simulink model "cartesian_trajectory_planner"  (R2020a)
settings: Solver=ode3  StartTime=0.0  StopTime=10  FixedStep=0.05  RelTol=1e-3
libraries: robotcorelib x2, robotmaniplib x2, simulink x1
settings Model: Creator=paolo  LastModifiedBy=paolo
settings OptimizationCC: EnhancedBackFolding=on  PassReuseOutputArgsAs=Individual arguments  ZeroExternalMemoryAtStartup=off  ZeroInternalMemoryAtStartup=off  MaxStackSize=64  OptimizeBlockOrder=speed  DifferentSizesBufferReuse=on  OptimizationCustomize=off  EfficientTunableParamExpr=on
settings DebuggingCC: ParameterTunabilityLossMsg=error
settings HardwareCC: ProdBitPerPointer=32  ProdBitPerSizeT=32  ProdBitPerPtrDiffT=32  ProdLargestAtomicFloat=None  ProdIntDivRoundTo=Undefined  ProdEndianess=Unspecified  ProdWordSize=32  ProdHWDeviceType=Generic->Unspecified (assume 32-bit Generic)
settings SFSimCC: MATLABDynamicMemAlloc=off
settings RTWCC: SystemTargetFile=ert.tlc  HardwareBoard=Robot Operating System (ROS)  TemplateMakefile=ert_default_tmf  Toolchain=Catkin  TargetLang=C++
settings CodeAppCC: ForceParamTrailComments=on  IgnoreCustomStorageClasses=off  OperatorAnnotations=on  SimulinkDataObjDesc=on  SFDataObjDesc=on  InsertBlockDesc=on

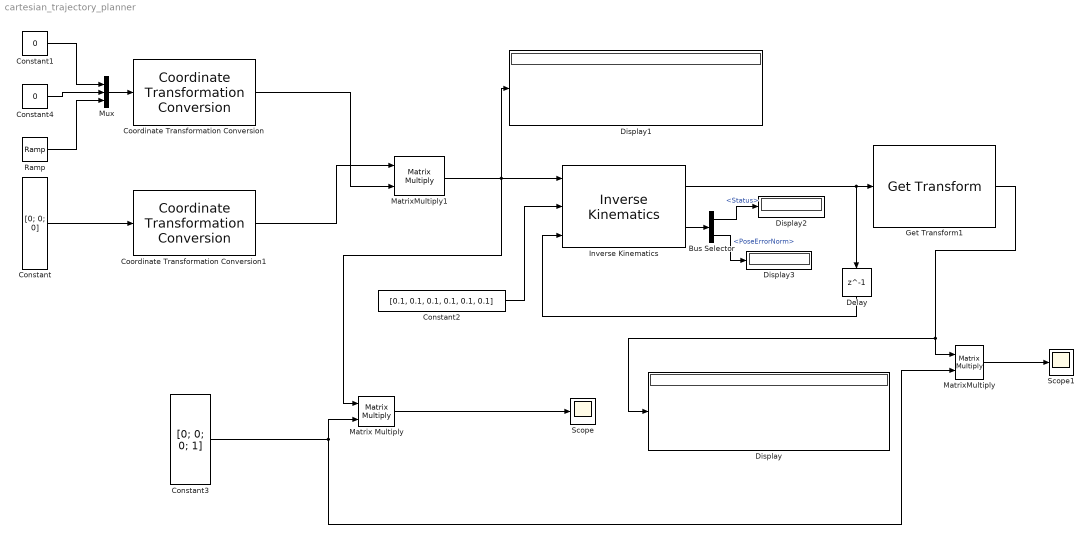
== system cartesian_trajectory_planner ==
  Bus Selector : BusSelector  OutputSignals=Status,PoseErrorNorm
  Constant : Constant  Value=[0; 0; 0]  VectorParams1D=off
  Constant1 : Constant  Value=0
  Constant2 : Constant  Value=[0.1, 0.1, 0.1, 0.1, 0.1, 0.1]
  Constant3 : Constant  Value=[0; 0; 0; 1]  VectorParams1D=off
  Constant4 : Constant  Value=0
  Coordinate Transformation Conversion : robotcorelib/Coordinate Transformation Conversion  InputRepresentation=Translation Vector  InputEulerSequence=ZYX  ShowTrVecInputPort=on  OutputRepresentation=Homogeneous Transformation  OutputEulerSequence=ZYX  ShowTrVecOutputPort=on  SimulateUsing=Interpreted execution
      settings: SourceProductBaseCode=NV,RO,RR
  Coordinate Transformation Conversion1 : robotcorelib/Coordinate Transformation Conversion  InputRepresentation=Euler Angles  InputEulerSequence=XYZ  ShowTrVecInputPort=off  OutputRepresentation=Homogeneous Transformation  OutputEulerSequence=ZYX  ShowTrVecOutputPort=on  SimulateUsing=Interpreted execution
      settings: SourceProductBaseCode=NV,RO,RR
  Delay : Delay  DelayLength=1  InitialCondition=[0; 0; 0; 0; 0; 0]
  Display{,1..3} (4 alike) : Display
  Get Transform1 : robotmaniplib/Get Transform  RigidBodyTree=robot  SourceBody=edo_link_ee  TargetBody=world  SimulateUsing=Interpreted execution
  Inverse Kinematics : robotmaniplib/Inverse Kinematics  RigidBodyTree=robot  EndEffector=edo_link_ee  ShowInfo=on  SolverName=BFGS Gradient Projection  EnforceJointLimits=on  MaxIterations=1500  MaxTime=10  GradientTolerance=1e-7  SolutionTolerance=1e-6  StepTolerance=1e-14  ErrorChangeTolerance=1e-12  UseErrorDamping=on  DampingBias=0.0025  SimulateUsing=Interpreted execution
  Matrix Multiply : Product  Multiplication=Matrix(*)
  MatrixMultiply : Product  Multiplication=Matrix(*)
  MatrixMultiply1 : Product  Multiplication=Matrix(*)
  Mux : Mux  Inputs=3
  Ramp : simulink/Sources/Ramp  slope=-0.01  start=0  InitialOutput=0.99
  Scope : Scope
  Scope1 : Scope
  wires:
  Constant2/1 -> Inverse Kinematics/2
  Inverse Kinematics/1 -> Get Transform1/1, Delay/1
  Delay/1 -> Inverse Kinematics/3
  Matrix Multiply/1 -> Scope/1
  Constant3/1 -> MatrixMultiply/2, Matrix Multiply/2
  MatrixMultiply/1 -> Scope1/1
  Get Transform1/1 -> Display/1, MatrixMultiply/1
  Mux/1 -> Coordinate Transformation Conversion/1
  Constant1/1 -> Mux/1
  Constant4/1 -> Mux/2
  Ramp/1 -> Mux/3
  Constant/1 -> Coordinate Transformation Conversion1/1
  Coordinate Transformation Conversion1/1 -> MatrixMultiply1/1
  Coordinate Transformation Conversion/1 -> MatrixMultiply1/2
  MatrixMultiply1/1 -> Display1/1, Matrix Multiply/1, Inverse Kinematics/1
  Inverse Kinematics/2 -> Bus Selector/1
  Bus Selector/1 -> Display2/1  "<Status>"
  Bus Selector/2 -> Display3/1  "<PoseErrorNorm>"
